simulink model "P_I_PI_Controller"  (R2021a)
settings: Solver=VariableStepAuto  StartTime=0.0  StopTime=20  MaxStep=1e-3  RelTol=1e-3
settings Model: Creator=lenovo  LastModifiedBy=lenovo

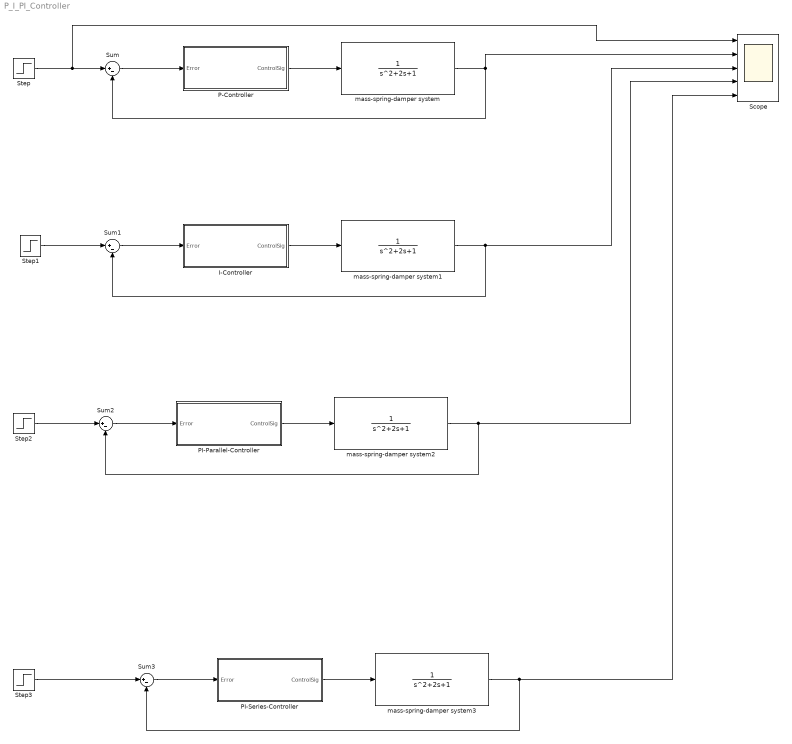
== system P_I_PI_Controller ==
   mass-spring-damper system{,1..3} (4 alike) : TransferFcn
  I-Controller : Subsystem
  P-Controller : Subsystem
  PI-Parallel-Controller : Subsystem
  PI-Series-Controller : Subsystem
  Scope : Scope  NumInputPorts=5
  Step{,1..3} (4 alike) : Step  SampleTime=0
  Sum{,1..3} (4 alike) : Sum  Inputs=|+-
  wires:
  P-Controller/1(ControlSig) -> " mass-spring-damper system"/1
  Sum/1 -> P-Controller/1(Error)
  " mass-spring-damper system"/1 -> Sum/2, Scope/2
  Step/1 -> Scope/1, Sum/1
  " mass-spring-damper system1"/1 -> Scope/3, Sum1/2
  Sum1/1 -> I-Controller/1(Error)
  I-Controller/1(ControlSig) -> " mass-spring-damper system1"/1
  Step1/1 -> Sum1/1
  Step2/1 -> Sum2/1
  PI-Parallel-Controller/1(ControlSig) -> " mass-spring-damper system2"/1
  Sum2/1 -> PI-Parallel-Controller/1(Error)
  " mass-spring-damper system2"/1 -> Sum2/2, Scope/4
  " mass-spring-damper system3"/1 -> Scope/5, Sum3/2
  Sum3/1 -> PI-Series-Controller/1(Error)
  PI-Series-Controller/1(ControlSig) -> " mass-spring-damper system3"/1
  Step3/1 -> Sum3/1

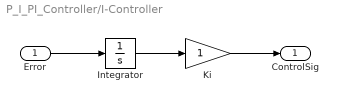
== system P_I_PI_Controller/I-Controller ==
  Error : Inport
  Integrator : Integrator
  Ki : Gain
  ControlSig : Outport
  wires:
  Ki/1 -> ControlSig/1
  Error/1 -> Integrator/1
  Integrator/1 -> Ki/1

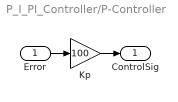
== system P_I_PI_Controller/P-Controller ==
  Error : Inport
  Kp : Gain  Gain=100
  ControlSig : Outport
  wires:
  Kp/1 -> ControlSig/1
  Error/1 -> Kp/1

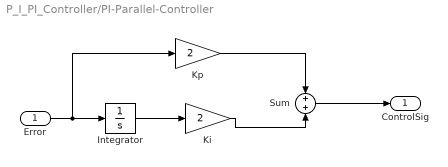
== system P_I_PI_Controller/PI-Parallel-Controller ==
  Error : Inport
  Integrator : Integrator
  Ki : Gain  Gain=2
  Kp : Gain  Gain=2
  Sum : Sum
  ControlSig : Outport
  wires:
  Integrator/1 -> Ki/1
  Error/1 -> Kp/1, Integrator/1
  Kp/1 -> Sum/1
  Ki/1 -> Sum/2
  Sum/1 -> ControlSig/1

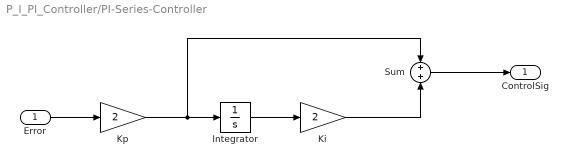
== system P_I_PI_Controller/PI-Series-Controller ==
  Error : Inport
  Integrator : Integrator
  Ki : Gain  Gain=2
  Kp : Gain  Gain=2
  Sum : Sum
  ControlSig : Outport
  wires:
  Sum/1 -> ControlSig/1
  Ki/1 -> Sum/2
  Kp/1 -> Sum/1, Integrator/1
  Error/1 -> Kp/1
  Integrator/1 -> Ki/1
